simulink model "exp_CLRC_DDF"  (R2024a)
settings: Solver=FixedStepDiscrete  StartTime=0.0  StopTime=inf  FixedStep=0.001  RelTol=1e-3  EnableMultiTasking=on
PreLoadFcn:
  | set_param(gcs, 'RTWSystemTargetFile', 'franka_emika_panda.tlc');
  | demos_common_configs();
values from neighbouring files (symbols this model uses):
  alpha = 75    [Panda_run.m]
  diff_alpha1 = 75    [Panda_run.m]
  GammaW = 0.2*eye(N)    [Panda_run.m]
  kapa1 = 1    [Panda_run.m]
  kapa2 = 0    [Panda_run.m]
  Kc = diag([20,20,20,20,8,8,5])    [Panda_run.m]
  Lambda = 10*eye(7)    [Panda_run.m]
  P0 = 0.2    [Panda_run.m]
  P1 = 1    [Panda_run.m]
  q0 = [0, -0.60, 0, -2.25, 0, 1.5, 0.8]'    [Panda_run.m]
  q1 = traj_c.qd.Data(:,1,1)    [Panda_run.m]
  robot_par = [basepar;fricpar]    [Panda_run.m]
  taud = 23    [Panda_run.m]
  Ts = 0.001    [Panda_run.m]
  vari = SD^2    (= 0)    [Panda_run.m]
undefined symbols (not defined in the file or in its folder): DiscIntNeverNeededParam
libraries: franka_simulink_library x8, matrix_library x2
settings Model: SimulationMode=external  ExtModeTrigDuration=10000  Creator=vasi_ko  LastModifiedBy=SYSU-RCLLab-G
settings SolverCC: AlgebraicLoopSolver=TrustRegion
settings DataIOCC: LimitDataPoints=on  SaveFormat=Array  ReturnWorkspaceOutputs=off
settings OptimizationCC: DefaultParameterBehavior=Inlined  EnhancedBackFolding=on  PassReuseOutputArgsThreshold=0  OptimizeBlockOrder=speed  DifferentSizesBufferReuse=on  OptimizationCustomize=off
settings DebuggingCC: SolverPrmCheckMsg=warning  ParameterTunabilityLossMsg=error  UnconnectedInputMsg=warning  UnconnectedOutputMsg=warning  UnconnectedLineMsg=warning  SFUnexpectedBacktrackingDiag=warning  SFNoUnconditionalDefaultTransitionDiag=warning  SFExecutionAtInitializationDiag=none  ArithmeticOperatorsInVariantConditions=warning
settings ModelReferenceCC: EnableRefExpFcnMdlSchedulingChecks=on  PropagateSignalLabelsOutOfModel=off
settings SFSimCC: SimUseLocalCustomCode=off  MATLABDynamicMemAlloc=off  CustomCodeUndefinedFunction=UseInterfaceOnly  SimTargetLang=C++
settings RTWCC: SystemTargetFile=franka_emika_panda.tlc  RTWVerbose=off  RTWUseLocalCustomCode=off  Toolchain=Franka Simulink | gmake (64-bit linux)  BuildConfiguration=Faster Runs  TargetLang=C++  GPUComputeCapability=3.5  DLArmComputeVersion=19.05
settings CodeAppCC: ForceParamTrailComments=on  OperatorAnnotations=on
settings STFCustomTargetCC: ModelReferenceCompliant=off  MatFileLogging=on  UseToolchainInfoCompliant=off  SystemTargetFile=franka_emika_panda.tlc
settings GRTTargetCC: ModelReferenceCompliant=off  ParMdlRefBuildCompliant=off  CompOptLevelCompliant=off  ConcurrentExecutionCompliant=off  CombineOutputUpdateFcns=off  CPPClassGenCompliant=off  GRTInterface=on  UseToolchainInfoCompliant=off  ExtModeStaticAlloc=on  ExtModeTransport=1  ExtModeMexFile=ext_xcp  ExtModeIntrfLevel=Level2 - Open
settings ConfigComp: CovMetricSettings=dw  CovSaveCumulativeToWorkspaceVar=on  CovSaveSingleToWorkspaceVar=on  CovExternalEMLEnable=off  CovSFcnEnable=off

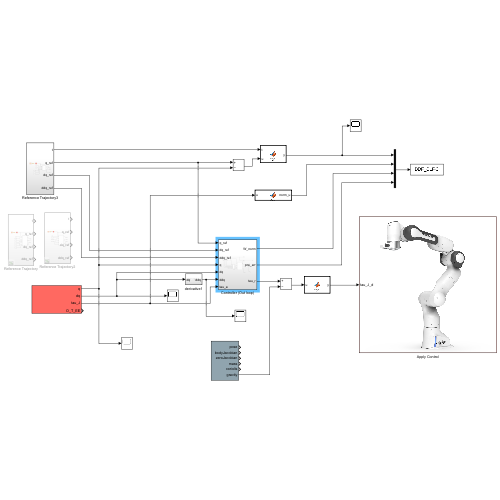
[thumbnail: Simulink's stored preview of the top-level diagram]
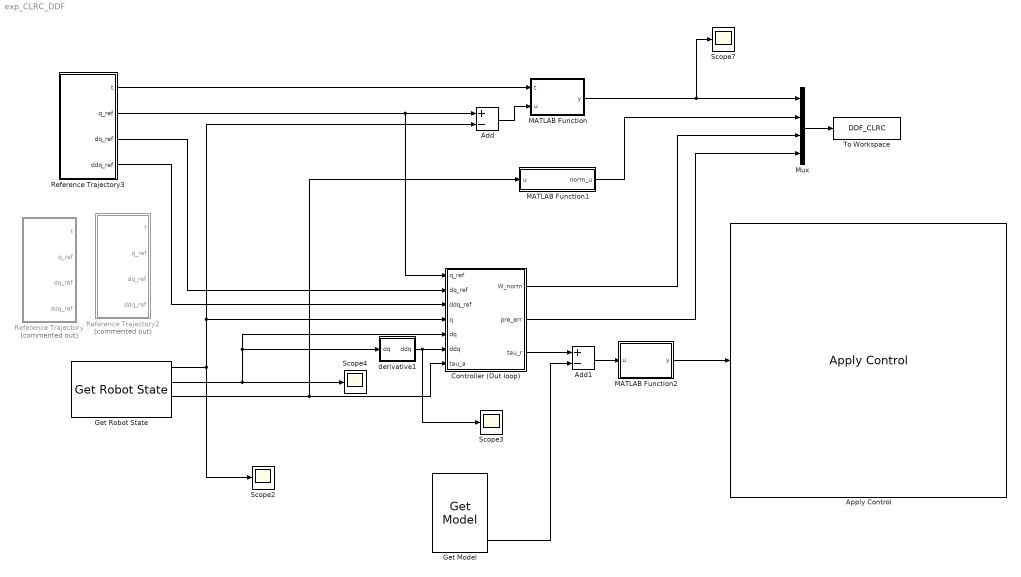
== system exp_CLRC_DDF ==
  Add : Sum  Inputs=+-
  Add1 : Sum  Inputs=+-
  Apply Control : franka_simulink_library/Apply Control  robot_ip=robot_ip  gripper_attached=off  control_mode=Torque Control  controller_choice=Joint Impedance Controller  elbow_control=on  collision_thresholds=collision_behavior  joint_impedance=joint_impedance  cartesian_impedance=cartesian_impedance  load_inertia=load_inertia  EE_T_K=EE_T_K  init_joint_configuration_req=on  init_joint_configuration=q0'
      settings: SourceProductName=Franka Emika Simulink Support Package
  Controller (Out loop) : Subsystem  SystemSampleTime=1e-3
  Get Model : franka_simulink_library/Get Model  robot_ip=robot_ip
      settings: SourceProductName=Franka Emika Simulink Support Package
  Get Robot State : franka_simulink_library/Get Robot State  robot_ip=robot_ip  signals_requested='q dq tau_J O_T_EE'
      settings: SourceProductName=Franka Emika Simulink Support Package
  MATLAB Function : MATLAB Function  TreatAsAtomicUnit=on
  MATLAB Function1 : MATLAB Function  TreatAsAtomicUnit=on
  MATLAB Function2 : MATLAB Function  TreatAsAtomicUnit=on
  Mux : Mux
  Reference Trajectory : Subsystem  Commented=on
  Reference Trajectory2 : Subsystem  Commented=on
  Reference Trajectory3 : Subsystem
  Scope{2..4,7} (4 alike) : Scope
  To Workspace : ToWorkspace  VariableName=DDF_CLRC  SampleTime=Ts
      settings: Save2DSignal=2-D array (concatenate along first dimension)
  derivative1 : Subsystem
  wires:
  Get Robot State/2 -> Scope4/1, Controller (Out loop)/5(dq), derivative1/1(dq)
  Add1/1 -> MATLAB Function2/1(u)
  Add/1 -> MATLAB Function/2(u)
  MATLAB Function/1(y) -> Scope7/1, Mux/1
  Get Robot State/3 -> MATLAB Function1/1(u), Controller (Out loop)/7(tau_a)
  Get Robot State/1 -> Scope2/1, Add/2, Controller (Out loop)/4(q)
  Reference Trajectory3/2(q_ref) -> Controller (Out loop)/1(q_ref), Add/1
  Reference Trajectory3/3(dq_ref) -> Controller (Out loop)/2(dq_ref)
  Reference Trajectory3/4(ddq_ref) -> Controller (Out loop)/3(ddq_ref)
  derivative1/1(ddq) -> Scope3/1, Controller (Out loop)/6(ddq)
  Controller (Out loop)/3(tau_r) -> Add1/1
  Get Model/6 -> Add1/2
  MATLAB Function2/1(y) -> Apply Control/1
  Reference Trajectory3/1(t) -> MATLAB Function/1(t)
  Mux/1 -> To Workspace/1
  MATLAB Function1/1(norm_u) -> Mux/2
  Controller (Out loop)/1(W_norm) -> Mux/3
  Controller (Out loop)/2(pre_err) -> Mux/4

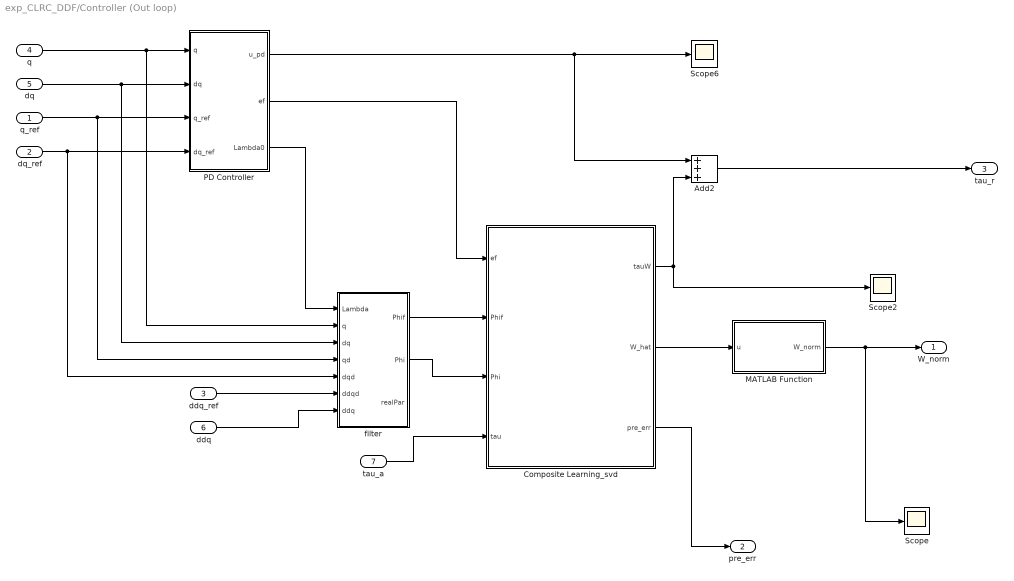
== system exp_CLRC_DDF/Controller (Out loop) ==
  q_ref : Inport
  dq_ref : Inport  Port=2
  ddq_ref : Inport  Port=3
  q : Inport  Port=4
  dq : Inport  Port=5
  ddq : Inport  Port=6
  tau_a : Inport  Port=7
  Add2 : Sum  Inputs=+++
  Composite Learning_svd : Subsystem
  MATLAB Function : MATLAB Function  TreatAsAtomicUnit=on
  PD Controller : Subsystem
  Scope : Scope
  Scope2 : Scope
  Scope6 : Scope
  filter : Subsystem
  W_norm : Outport
  pre_err : Outport  Port=2
  tau_r : Outport  Port=3
  wires:
  q_ref/1 -> PD Controller/3(q_ref), filter/4(qd)
  dq_ref/1 -> PD Controller/4(dq_ref), filter/5(dqd)
  dq/1 -> filter/3(dq), PD Controller/2(dq)
  PD Controller/1(u_pd) -> Scope6/1, Add2/1
  ddq_ref/1 -> filter/6(ddqd)
  Composite Learning_svd/2(W_hat) -> MATLAB Function/1(u)
  MATLAB Function/1(W_norm) -> Scope/1, W_norm/1
  filter/1(Phif) -> Composite Learning_svd/2(Phif)
  filter/2(Phi) -> Composite Learning_svd/3(Phi)
  PD Controller/2(ef) -> Composite Learning_svd/1(ef)
  Composite Learning_svd/1(tauW) -> Scope2/1, Add2/3
  ddq/1 -> filter/7(ddq)
  q/1 -> PD Controller/1(q), filter/2(q)
  Add2/1 -> tau_r/1
  tau_a/1 -> Composite Learning_svd/4(tau)
  PD Controller/3(Lambda0) -> filter/1(Lambda)
  Composite Learning_svd/3(pre_err) -> pre_err/1

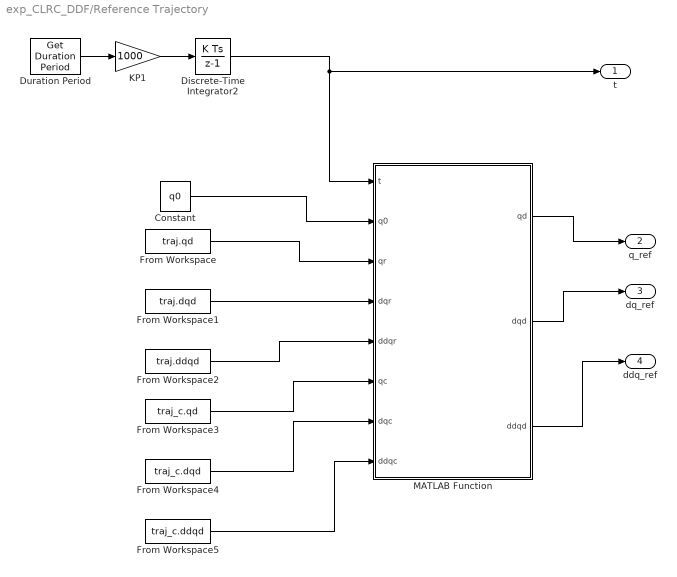
== system exp_CLRC_DDF/Reference Trajectory ==
  Constant : Constant  Value=q0
  Discrete-Time Integrator2 : DiscreteIntegrator  SampleTime=-1  ICPrevOutput=DiscIntNeverNeededParam  ICPrevScaledInput=DiscIntNeverNeededParam
  Duration Period : franka_simulink_library/Get Duration Period  robot_ip=robot_ip
      settings: SourceProductName=Franka Emika Simulink Support Package
  From Workspace : FromWorkspace  VariableName=traj.qd
  From Workspace1 : FromWorkspace  VariableName=traj.dqd
  From Workspace2 : FromWorkspace  VariableName=traj.ddqd
  From Workspace3 : FromWorkspace  VariableName=traj_c.qd
  From Workspace4 : FromWorkspace  VariableName=traj_c.dqd
  From Workspace5 : FromWorkspace  VariableName=traj_c.ddqd
  KP1 : Gain  Gain=1000
  MATLAB Function : MATLAB Function  TreatAsAtomicUnit=on
  t : Outport
  q_ref : Outport  Port=2
  dq_ref : Outport  Port=3
  ddq_ref : Outport  Port=4
  wires:
  From Workspace/1 -> MATLAB Function/3(qr)
  From Workspace1/1 -> MATLAB Function/4(dqr)
  From Workspace2/1 -> MATLAB Function/5(ddqr)
  Discrete-Time Integrator2/1 -> t/1, MATLAB Function/1(t)
  Constant/1 -> MATLAB Function/2(q0)
  MATLAB Function/1(qd) -> q_ref/1
  MATLAB Function/2(dqd) -> dq_ref/1
  MATLAB Function/3(ddqd) -> ddq_ref/1
  KP1/1 -> Discrete-Time Integrator2/1
  Duration Period/1 -> KP1/1
  From Workspace3/1 -> MATLAB Function/6(qc)
  From Workspace4/1 -> MATLAB Function/7(dqc)
  From Workspace5/1 -> MATLAB Function/8(ddqc)

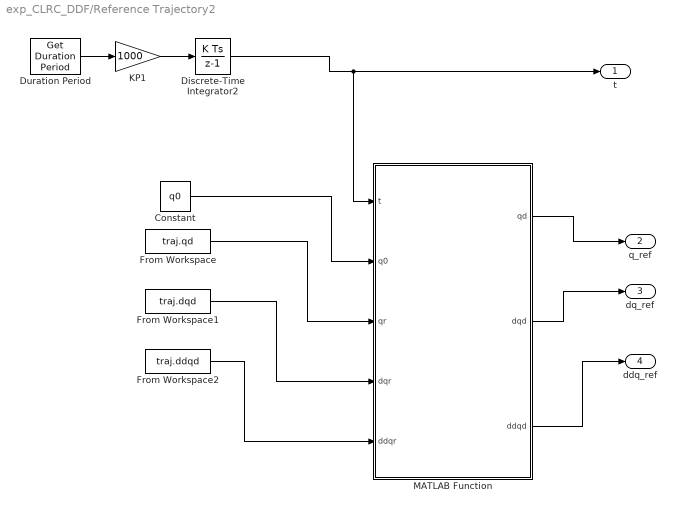
== system exp_CLRC_DDF/Reference Trajectory2 ==
  Constant : Constant  Value=q0
  Discrete-Time Integrator2 : DiscreteIntegrator  SampleTime=-1  ICPrevOutput=DiscIntNeverNeededParam  ICPrevScaledInput=DiscIntNeverNeededParam
  Duration Period : franka_simulink_library/Get Duration Period  robot_ip=robot_ip
      settings: SourceProductName=Franka Emika Simulink Support Package
  From Workspace : FromWorkspace  VariableName=traj.qd
  From Workspace1 : FromWorkspace  VariableName=traj.dqd
  From Workspace2 : FromWorkspace  VariableName=traj.ddqd
  KP1 : Gain  Gain=1000
  MATLAB Function : MATLAB Function  TreatAsAtomicUnit=on
  t : Outport
  q_ref : Outport  Port=2
  dq_ref : Outport  Port=3
  ddq_ref : Outport  Port=4
  wires:
  From Workspace/1 -> MATLAB Function/3(qr)
  From Workspace1/1 -> MATLAB Function/4(dqr)
  From Workspace2/1 -> MATLAB Function/5(ddqr)
  Discrete-Time Integrator2/1 -> t/1, MATLAB Function/1(t)
  Constant/1 -> MATLAB Function/2(q0)
  MATLAB Function/1(qd) -> q_ref/1
  MATLAB Function/2(dqd) -> dq_ref/1
  MATLAB Function/3(ddqd) -> ddq_ref/1
  KP1/1 -> Discrete-Time Integrator2/1
  Duration Period/1 -> KP1/1

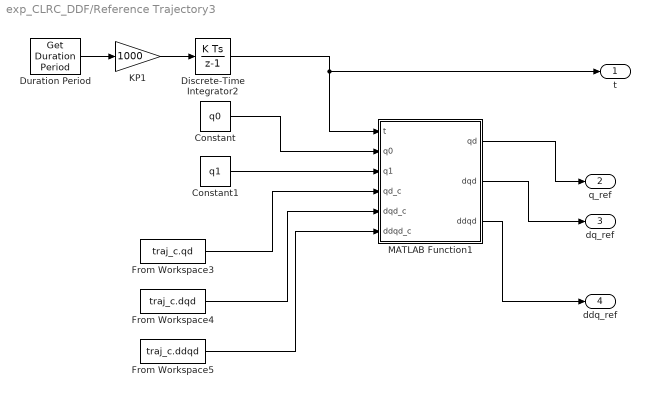
== system exp_CLRC_DDF/Reference Trajectory3 ==
  Constant : Constant  Value=q0
  Constant1 : Constant  Value=q1
  Discrete-Time Integrator2 : DiscreteIntegrator  SampleTime=-1  ICPrevOutput=DiscIntNeverNeededParam  ICPrevScaledInput=DiscIntNeverNeededParam
  Duration Period : franka_simulink_library/Get Duration Period  robot_ip=robot_ip
      settings: SourceProductName=Franka Emika Simulink Support Package
  From Workspace3 : FromWorkspace  VariableName=traj_c.qd
  From Workspace4 : FromWorkspace  VariableName=traj_c.dqd
  From Workspace5 : FromWorkspace  VariableName=traj_c.ddqd
  KP1 : Gain  Gain=1000
  MATLAB Function1 : MATLAB Function  TreatAsAtomicUnit=on
  t : Outport
  q_ref : Outport  Port=2
  dq_ref : Outport  Port=3
  ddq_ref : Outport  Port=4
  wires:
  MATLAB Function1/1(qd) -> q_ref/1
  MATLAB Function1/2(dqd) -> dq_ref/1
  MATLAB Function1/3(ddqd) -> ddq_ref/1
  From Workspace3/1 -> MATLAB Function1/4(qd_c)
  From Workspace4/1 -> MATLAB Function1/5(dqd_c)
  From Workspace5/1 -> MATLAB Function1/6(ddqd_c)
  KP1/1 -> Discrete-Time Integrator2/1
  Duration Period/1 -> KP1/1
  Discrete-Time Integrator2/1 -> MATLAB Function1/1(t), t/1
  Constant/1 -> MATLAB Function1/2(q0)
  Constant1/1 -> MATLAB Function1/3(q1)

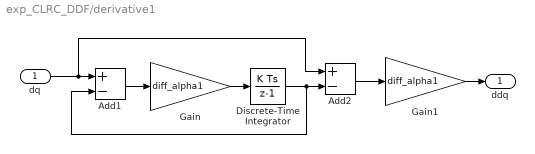
== system exp_CLRC_DDF/derivative1 ==
  dq : Inport
  Add1 : Sum  Inputs=+-
  Add2 : Sum  Inputs=+-
  Discrete-Time Integrator : DiscreteIntegrator  SampleTime=-1  ICPrevOutput=DiscIntNeverNeededParam  ICPrevScaledInput=DiscIntNeverNeededParam
  Gain : Gain  Gain=diff_alpha1
  Gain1 : Gain  Gain=diff_alpha1
  ddq : Outport
  wires:
  Gain/1 -> Discrete-Time Integrator/1
  Add1/1 -> Gain/1
  dq/1 -> Add2/1, Add1/1
  Add2/1 -> Gain1/1
  Discrete-Time Integrator/1 -> Add2/2, Add1/2
  Gain1/1 -> ddq/1

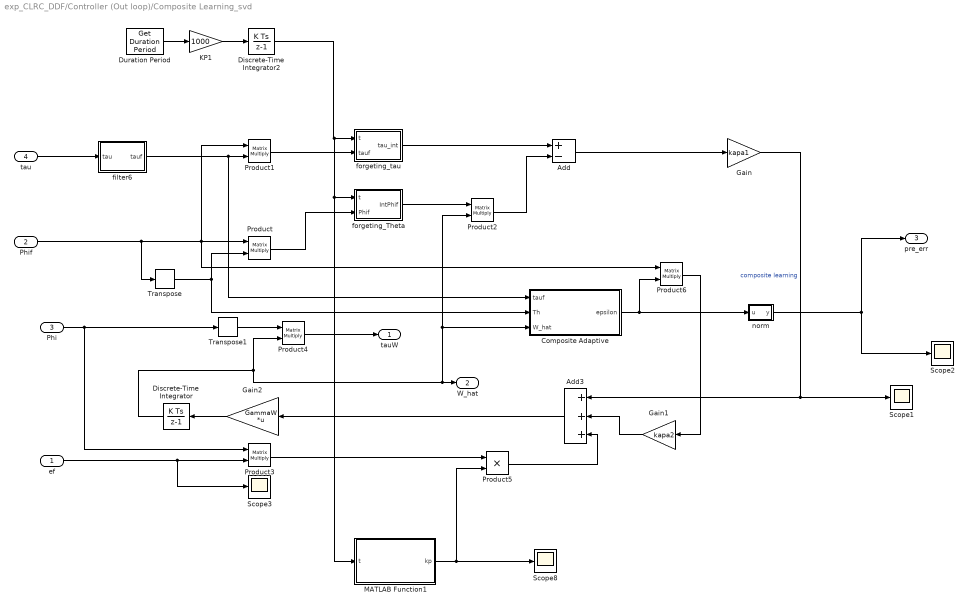
== system exp_CLRC_DDF/Controller (Out loop)/Composite Learning_svd ==
  ef : Inport
  Phif : Inport  Port=2
  Phi : Inport  Port=3
  tau : Inport  Port=4
  Add : Sum  Inputs=+-
  Add3 : Sum  Inputs=+++
  Composite Adaptive : Subsystem
  Discrete-Time Integrator : DiscreteIntegrator  SampleTime=-1  ICPrevOutput=DiscIntNeverNeededParam  ICPrevScaledInput=DiscIntNeverNeededParam
  Discrete-Time Integrator2 : DiscreteIntegrator  SampleTime=-1  ICPrevOutput=DiscIntNeverNeededParam  ICPrevScaledInput=DiscIntNeverNeededParam
  Duration Period : franka_simulink_library/Get Duration Period  robot_ip=robot_ip
      settings: SourceProductName=Franka Emika Simulink Support Package
  Gain : Gain  Gain=kapa1
  Gain1 : Gain  Gain=kapa2
  Gain2 : Gain  Gain=GammaW  Multiplication=Matrix(K*u)
  KP1 : Gain  Gain=1000
  MATLAB Function1 : MATLAB Function  TreatAsAtomicUnit=on
  Product{,1..4,6} (6 alike) : Product  Multiplication=Matrix(*)
  Product5 : Product
  Scope{1..3,8} (4 alike) : Scope
  Transpose : matrix_library/Transpose
  Transpose1 : matrix_library/Transpose
  filter6 : Subsystem
  forgeting_Theta : Subsystem
  forgeting_tau : Subsystem
  norm : MATLAB Function  TreatAsAtomicUnit=on
  tauW : Outport
  W_hat : Outport  Port=2
  pre_err : Outport  Port=3
  wires:
  Transpose/1 -> Composite Adaptive/2(Th), Product/2
  ef/1 -> Scope3/1, Product3/2
  Phi/1 -> Transpose1/1, Product3/1
  Transpose1/1 -> Product4/1
  Gain2/1 -> Discrete-Time Integrator/1
  Add3/1 -> Gain2/1
  Product6/1 -> Gain1/1
  Product4/1 -> tauW/1
  norm/1(y) -> Scope2/1, pre_err/1
  Product3/1 -> Product5/1
  Gain/1 -> Add3/1, Scope1/1  "composite learning"
  Discrete-Time Integrator/1 -> Product2/2, Composite Adaptive/3(W_hat), W_hat/1, Product4/2
  Product/1 -> forgeting_Theta/2(Phif)
  Product1/1 -> forgeting_tau/2(tauf)
  forgeting_Theta/1(IntPhif) -> Product2/1
  forgeting_tau/1(tau_int) -> Add/1
  Product2/1 -> Add/2
  Add/1 -> Gain/1
  KP1/1 -> Discrete-Time Integrator2/1
  Duration Period/1 -> KP1/1
  Discrete-Time Integrator2/1 -> MATLAB Function1/1(t), forgeting_Theta/1(t), forgeting_tau/1(t)
  MATLAB Function1/1(kp) -> Scope8/1, Product5/2
  Product5/1 -> Add3/3
  Composite Adaptive/1(epsilon) -> Product6/2, norm/1(u)
  Phif/1 -> Product1/1, Product6/1, Product/1, Transpose/1
  Gain1/1 -> Add3/2
  tau/1 -> filter6/1(tau)
  filter6/1(tauf) -> Composite Adaptive/1(tauf), Product1/2

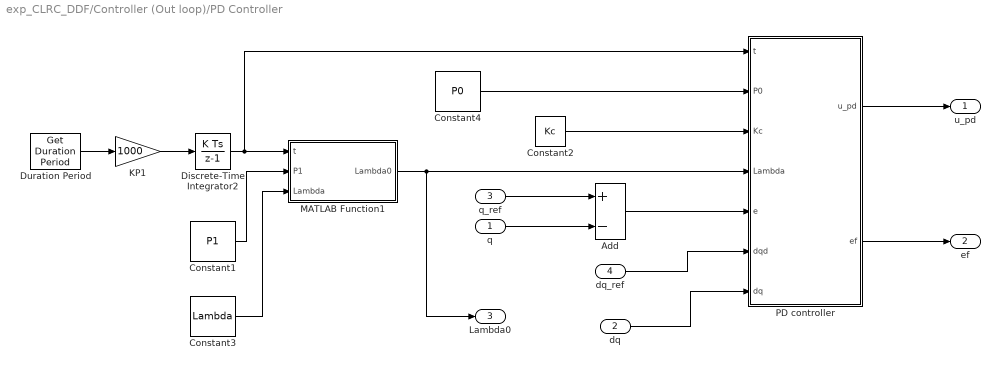
== system exp_CLRC_DDF/Controller (Out loop)/PD Controller ==
  q : Inport
  dq : Inport  Port=2
  q_ref : Inport  Port=3
  dq_ref : Inport  Port=4
  Add : Sum  Inputs=+-
  Constant1 : Constant  Value=P1
  Constant2 : Constant  Value=Kc
  Constant3 : Constant  Value=Lambda
  Constant4 : Constant  Value=P0
  Discrete-Time Integrator2 : DiscreteIntegrator  SampleTime=-1  ICPrevOutput=DiscIntNeverNeededParam  ICPrevScaledInput=DiscIntNeverNeededParam
  Duration Period : franka_simulink_library/Get Duration Period  robot_ip=robot_ip
      settings: SourceProductName=Franka Emika Simulink Support Package
  KP1 : Gain  Gain=1000
  MATLAB Function1 : MATLAB Function  TreatAsAtomicUnit=on
  PD controller : MATLAB Function  TreatAsAtomicUnit=on
  u_pd : Outport
  ef : Outport  Port=2
  Lambda0 : Outport  Port=3
  wires:
  Duration Period/1 -> KP1/1
  Constant2/1 -> PD controller/3(Kc)
  q/1 -> Add/2
  MATLAB Function1/1(Lambda0) -> Lambda0/1, PD controller/4(Lambda)
  KP1/1 -> Discrete-Time Integrator2/1
  Discrete-Time Integrator2/1 -> PD controller/1(t), MATLAB Function1/1(t)
  Constant3/1 -> MATLAB Function1/3(Lambda)
  Add/1 -> PD controller/5(e)
  q_ref/1 -> Add/1
  PD controller/1(u_pd) -> u_pd/1
  PD controller/2(ef) -> ef/1
  Constant1/1 -> MATLAB Function1/2(P1)
  Constant4/1 -> PD controller/2(P0)
  dq_ref/1 -> PD controller/6(dqd)
  dq/1 -> PD controller/7(dq)

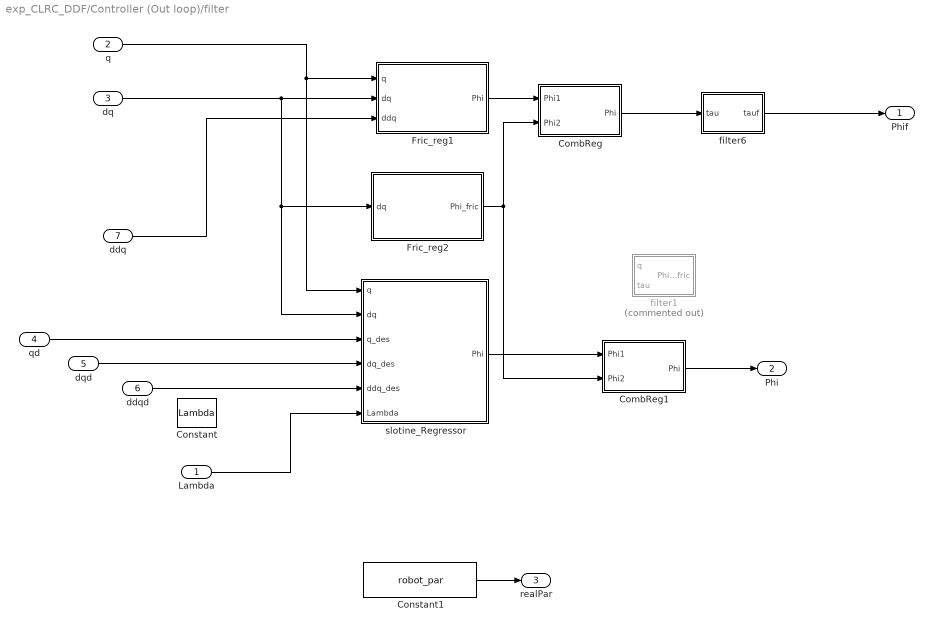
== system exp_CLRC_DDF/Controller (Out loop)/filter ==
  Lambda : Inport
  q : Inport  Port=2
  dq : Inport  Port=3
  qd : Inport  Port=4
  dqd : Inport  Port=5
  ddqd : Inport  Port=6
  ddq : Inport  Port=7
  CombReg : MATLAB Function  TreatAsAtomicUnit=on
  CombReg1 : MATLAB Function  TreatAsAtomicUnit=on
  Constant : Constant  Value=Lambda
  Constant1 : Constant  Value=robot_par
  Fric_reg1 : MATLAB Function  TreatAsAtomicUnit=on
  Fric_reg2 : MATLAB Function  TreatAsAtomicUnit=on
  filter1 : Subsystem  Commented=on
  filter6 : Subsystem
  slotine_Regressor : MATLAB Function  TreatAsAtomicUnit=on
  Phif : Outport
  Phi : Outport  Port=2
  realPar : Outport  Port=3
  wires:
  qd/1 -> slotine_Regressor/3(q_des)
  dqd/1 -> slotine_Regressor/4(dq_des)
  ddqd/1 -> slotine_Regressor/5(ddq_des)
  Lambda/1 -> slotine_Regressor/6(Lambda)
  dq/1 -> Fric_reg2/1(dq), slotine_Regressor/2(dq), Fric_reg1/2(dq)
  slotine_Regressor/1(Phi) -> CombReg1/1(Phi1)
  Constant1/1 -> realPar/1
  CombReg1/1(Phi) -> Phi/1
  ddq/1 -> Fric_reg1/3(ddq)
  q/1 -> Fric_reg1/1(q), slotine_Regressor/1(q)
  Fric_reg1/1(Phi) -> CombReg/1(Phi1)
  Fric_reg2/1(Phi_fric) -> CombReg/2(Phi2), CombReg1/2(Phi2)
  CombReg/1(Phi) -> filter6/1(tau)
  filter6/1(tauf) -> Phif/1

== system exp_CLRC_DDF/Controller (Out loop)/Composite Learning_svd/Composite Adaptive ==
  tauf : Inport
  Th : Inport  Port=2
  W_hat : Inport  Port=3
  Add1 : Sum  Inputs=+-
  Product6 : Product  Multiplication=Matrix(*)
  epsilon : Outport
  wires:
  Add1/1 -> epsilon/1
  Product6/1 -> Add1/2
  tauf/1 -> Add1/1
  Th/1 -> Product6/1
  W_hat/1 -> Product6/2

== system exp_CLRC_DDF/Controller (Out loop)/Composite Learning_svd/filter6 ==
  tau : Inport
  Add : Sum  Inputs=++-
  Discrete-Time Integrator : DiscreteIntegrator  SampleTime=-1  ICPrevOutput=DiscIntNeverNeededParam  ICPrevScaledInput=DiscIntNeverNeededParam
  Gain : Gain  Gain=alpha
  tauf : Outport
  wires:
  tau/1 -> Add/2
  Add/1 -> Gain/1
  Gain/1 -> Discrete-Time Integrator/1
  Discrete-Time Integrator/1 -> Add/3, tauf/1

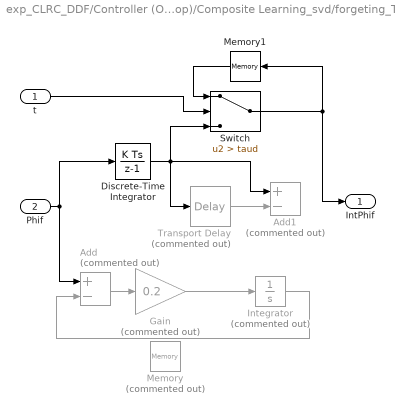
== system exp_CLRC_DDF/Controller (Out loop)/Composite Learning_svd/forgeting_Theta ==
  t : Inport
  Phif : Inport  Port=2
  Add : Sum  Commented=on  Inputs=+-
  Add1 : Sum  Commented=on  Inputs=+-
  Discrete-Time Integrator : DiscreteIntegrator  SampleTime=-1  ICPrevOutput=DiscIntNeverNeededParam  ICPrevScaledInput=DiscIntNeverNeededParam
  Gain : Gain  Commented=on  Gain=0.2
  Integrator : Integrator  Commented=on  UpperSaturationLimit=20  LowerSaturationLimit=-20
  Memory : Memory  Commented=on
  Memory1 : Memory
  Switch : Switch  Criteria=u2 > Threshold  Threshold=taud  SaturateOnIntegerOverflow=off  InputSameDT=off
  Transport Delay : TransportDelay  Commented=on  DelayTime=taud  BufferSize=taud/Ts
  IntPhif : Outport
  wires:
  Gain/1 -> Integrator/1
  Add/1 -> Gain/1
  Integrator/1 -> Add/2
  t/1 -> Switch/2
  Phif/1 -> Discrete-Time Integrator/1, Add/1
  Memory1/1 -> Switch/1
  Discrete-Time Integrator/1 -> Switch/3, Add1/1, Transport Delay/1
  Transport Delay/1 -> Add1/2
  Switch/1 -> Memory1/1, IntPhif/1

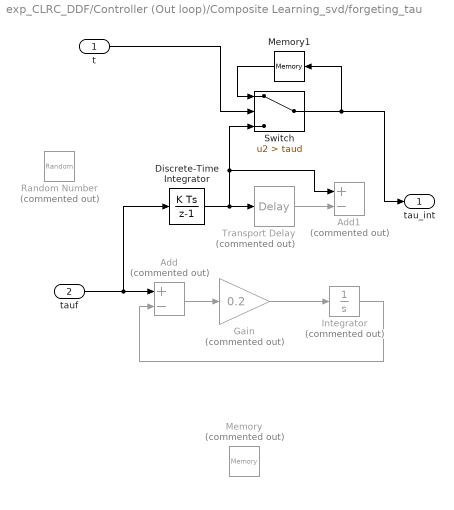
== system exp_CLRC_DDF/Controller (Out loop)/Composite Learning_svd/forgeting_tau ==
  t : Inport
  tauf : Inport  Port=2
  Add : Sum  Commented=on  Inputs=+-
  Add1 : Sum  Commented=on  Inputs=+-
  Discrete-Time Integrator : DiscreteIntegrator  SampleTime=-1  ICPrevOutput=DiscIntNeverNeededParam  ICPrevScaledInput=DiscIntNeverNeededParam
  Gain : Gain  Commented=on  Gain=0.2
  Integrator : Integrator  Commented=on  UpperSaturationLimit=20  LowerSaturationLimit=-20
  Memory : Memory  Commented=on
  Memory1 : Memory
  Random Number : RandomNumber  Commented=on  Variance=vari  SampleTime=0.1
  Switch : Switch  Criteria=u2 > Threshold  Threshold=taud  SaturateOnIntegerOverflow=off  InputSameDT=off
  Transport Delay : TransportDelay  Commented=on  DelayTime=taud  BufferSize=taud/Ts
  tau_int : Outport
  wires:
  Gain/1 -> Integrator/1
  tauf/1 -> Discrete-Time Integrator/1, Add/1
  Add/1 -> Gain/1
  Integrator/1 -> Add/2
  Transport Delay/1 -> Add1/2
  t/1 -> Switch/2
  Discrete-Time Integrator/1 -> Switch/3, Add1/1, Transport Delay/1
  Memory1/1 -> Switch/1
  Switch/1 -> tau_int/1, Memory1/1

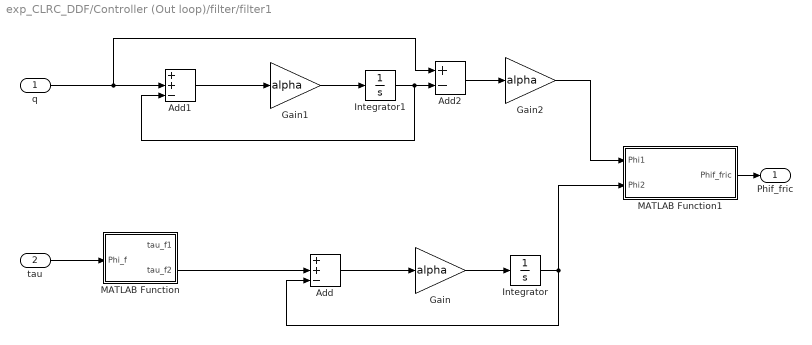
== system exp_CLRC_DDF/Controller (Out loop)/filter/filter1 ==
  q : Inport
  tau : Inport  Port=2
  Add : Sum  Inputs=++-
  Add1 : Sum  Inputs=++-
  Add2 : Sum  Inputs=+-
  Gain : Gain  Gain=alpha
  Gain1 : Gain  Gain=alpha
  Gain2 : Gain  Gain=alpha
  Integrator : Integrator  UpperSaturationLimit=20  LowerSaturationLimit=-20
  Integrator1 : Integrator  InitialCondition=q0  UpperSaturationLimit=20  LowerSaturationLimit=-20
  MATLAB Function : MATLAB Function  TreatAsAtomicUnit=on
  MATLAB Function1 : MATLAB Function  TreatAsAtomicUnit=on
  Phif_fric : Outport
  wires:
  Add/1 -> Gain/1
  Gain/1 -> Integrator/1
  Integrator/1 -> Add/3, MATLAB Function1/2(Phi2)
  tau/1 -> MATLAB Function/1(Phi_f)
  MATLAB Function/2(tau_f2) -> Add/2
  Integrator1/1 -> Add1/3, Add2/2
  Gain1/1 -> Integrator1/1
  Add1/1 -> Gain1/1
  q/1 -> Add2/1, Add1/2
  Add2/1 -> Gain2/1
  MATLAB Function1/1(Phif_fric) -> Phif_fric/1
  Gain2/1 -> MATLAB Function1/1(Phi1)

== system exp_CLRC_DDF/Controller (Out loop)/filter/filter6 ==
  tau : Inport
  Add : Sum  Inputs=++-
  Discrete-Time Integrator : DiscreteIntegrator  SampleTime=-1  ICPrevOutput=DiscIntNeverNeededParam  ICPrevScaledInput=DiscIntNeverNeededParam
  Gain : Gain  Gain=alpha
  tauf : Outport
  wires:
  tau/1 -> Add/2
  Add/1 -> Gain/1
  Gain/1 -> Discrete-Time Integrator/1
  Discrete-Time Integrator/1 -> Add/3, tauf/1

== matlab function exp_CLRC_DDF/Controller (Out loop)/Composite Learning_svd/norm ==
  data: u input; y output
function y= fcn(u)

y = norm(u);

== matlab function exp_CLRC_DDF/Controller (Out loop)/filter/CombReg ==
  data: Phi1 input; Phi output; Phi2 input
function Phi = fcn(Phi1,Phi2)

Phi = [Phi1;Phi2];

== matlab function exp_CLRC_DDF/Controller (Out loop)/filter/CombReg1 ==
  data: Phi1 input; Phi output; Phi2 input
function Phi = fcn(Phi1,Phi2)

Phi = [Phi1;Phi2];

== matlab function exp_CLRC_DDF/Reference Trajectory/MATLAB Function ==
  data: t input; q0 input; qd output; qr input; dqr input; ddqr input; dqd output; ddqd output; qc input; dqc input; ddqc input
function [qd,dqd,ddqd] = fcn(t,q0,qr,dqr,ddqr,qc,dqc,ddqc)

if t<=100
    qd=qr;dqd=dqr;ddqd=ddqr;
elseif t<=150
    qd=qc;dqd=dqc;ddqd=ddqc;
else
    qd=q0;dqd=zeros(7,1);ddqd=zeros(7,1);
end

== matlab function exp_CLRC_DDF/Controller (Out loop)/filter/filter1/MATLAB Function ==
  data: Phi_f input; tau_f1 output; tau_f2 output
function [tau_f1,tau_f2] = fcn(Phi_f)
tau_f1=Phi_f(1:7,:);
tau_f2 = Phi_f(8:end,:);

== matlab function exp_CLRC_DDF/Controller (Out loop)/filter/filter1/MATLAB Function1 ==
  data: Phi1 input; Phif_fric output; Phi2 input
function Phif_fric = fcn(Phi1,Phi2)
Phif_fric=[diag(Phi1);Phi2];

== matlab function exp_CLRC_DDF/Reference Trajectory2/MATLAB Function ==
  data: t input; q0 input; qd output; qr input; dqr input; ddqr input; dqd output; ddqd output
function [qd,dqd,ddqd] = fcn(t,q0,qr,dqr,ddqr)

if t<=140
    qd=qr;dqd=dqr;ddqd=ddqr;
else
    qd=q0;dqd=zeros(7,1);ddqd=zeros(7,1);
end

== matlab function exp_CLRC_DDF/MATLAB Function1 ==
  data: u input; norm_u output
function norm_u= fcn(u)

norm_u = norm(u);

== matlab function exp_CLRC_DDF/Controller (Out loop)/MATLAB Function ==
  data: u input; W_norm output
function W_norm= fcn(u)

W_norm = norm(u);

== matlab function exp_CLRC_DDF/Reference Trajectory3/MATLAB Function1 ==
  data: t input; q0 input; q1 input; qd output; dqd output; ddqd output; qd_c input; dqd_c input; ddqd_c input
function [qd,dqd,ddqd] = fcn(t,q0,q1,qd_c,dqd_c,ddqd_c)

if t<=100
    T=[0,3,6,9,13,17,20,23];
    P=[q0';
        -0.75, 0.25, 0, -0.8, -1.2, 0.5, -1.8;
        1.5, 0.6, -0.83, -0.5, 1.04, 1.6, -2.0;
        0.25, -0.55, 0.3, -1.75, 0.25, 0.75, 0.50;
        -1.20, 0.84, -0.85, -1.0, 1.07, 2.55, 2.05;
        -2.25, -1.2, 2.23, -0.63, -0.54, 2.8, 1.3;
        -0.25, 1.0, -0.23, -1.33, -0.24, 1.1, -2.5;
        q0'];
    [qd,dqd,ddqd]=traj_gen_fun(t,T,P);
elseif t<=120
    T=[100,105];
    P=[q0,q1]';
    [qd,dqd,ddqd]=traj_gen_fun(t,T,P);
elseif t<=160
    qd=qd_c;dqd=dqd_c;ddqd=ddqd_c;
else
    T=[160,165];
    P=[q1,q0]';
    [qd,dqd,ddqd]=traj_gen_fun(t,T,P);

    % qd=[0, -0.60, 0, -2.25, 0, 1.5, 0.8]';
    % dqd=zeros(7,1);
    % ddqd=zeros(7,1);
end

== matlab function exp_CLRC_DDF/Controller (Out loop)/filter/Fric_reg1 ==
  data: q input; dq input; Phi output; ddq input
function Phi = fcn(q,dq,ddq)

Phi = Base_Regressor_Panda(q,dq,ddq);

== matlab function exp_CLRC_DDF/Controller (Out loop)/filter/Fric_reg2 ==
  data: dq input; Phi_fric output
function Phi_fric = fcn(dq)

Phi_fric = Regressor_fric(dq);

== matlab function exp_CLRC_DDF/MATLAB Function2 ==
  data: u input; y output
function y = fcn(u)

y = u';

== matlab function exp_CLRC_DDF/MATLAB Function ==
  data: t input; u input; y output
function y = fcn(t,u)
if t==0
    u=zeros(7,1);
end
y = norm(u);

== matlab function exp_CLRC_DDF/Controller (Out loop)/filter/slotine_Regressor ==
  data: q input; Phi output; dq input; q_des input; dq_des input; ddq_des input; Lambda input
function Phi = fcn(q,dq,q_des,dq_des,ddq_des,Lambda)
e1=q-q_des;
de1=dq-dq_des;


dqr=(dq_des-Lambda*e1);

ddqr=ddq_des-Lambda*de1;

Phi=Base_Slotine_Panda(q,dq,dqr,ddqr);

== matlab function exp_CLRC_DDF/Controller (Out loop)/PD Controller/MATLAB Function1 ==
  data: t input; P1 input; Lambda0 output; Lambda input
function Lambda0= fcn(t,P1,Lambda)


%% Lambda
% P0=0.5;
if t<40
    Lambda0=Lambda;
elseif t<100
    Lambda0=Lambda-0.5*(1+tanh((t-70)/5))*(1-P1)*Lambda;
else
    Lambda0=P1*Lambda;
end

== matlab function exp_CLRC_DDF/Controller (Out loop)/Composite Learning_svd/MATLAB Function1 ==
  data: t input; kp output
function kp= fcn(t)


%% Lambda
% P0=0.5;

if t<40
    kp=1;
elseif t<100
    kp=1-0.5*(1+tanh((t-70)/5));
else
    kp=0;
end

== matlab function exp_CLRC_DDF/Controller (Out loop)/PD Controller/PD controller ==
  data: t input; P0 input; Kc input; Lambda input; e input; dqd input; u_pd output; dq input; ef output
function [u_pd,ef]= fcn(t,P0,Kc,Lambda,e,dqd,dq)
% 
dqr=(dqd+Lambda*e);

ef=dqr-dq;


%% Kc
% P0=0.2;
if t<40
    Kc0=Kc;
elseif t<100
    Kc0=Kc-0.5*(1+tanh((t-70)/5))*(1-P0)*Kc;
else
    Kc0=P0*Kc;
end


u_pd = Kc0*ef;
